simulink model "Controller_CalDistance0"  (R2020b)
settings: Solver=FixedStepDiscrete  StartTime=0.0  StopTime=inf  FixedStep=1e-06  RelTol=1e-3  EnableMultiTasking=on
settings Model: SILPILModeSetting=veronly  ExtModeTrigDuration=2  Creator=99714  LastModifiedBy=99714
settings DataIOCC: SaveOutput=off  SaveTime=off
settings OptimizationCC: EnhancedBackFolding=on  PassReuseOutputArgsAs=Individual arguments  MaxStackSize=64  OptimizeBlockOrder=speed  DifferentSizesBufferReuse=on  OptimizationCustomize=off  EfficientTunableParamExpr=on
settings DebuggingCC: ParameterTunabilityLossMsg=error
settings HardwareCC: ProdBitPerInt=16  ProdBitPerPointer=16  ProdBitPerSizeT=16  ProdBitPerPtrDiffT=16  ProdLargestAtomicFloat=None  ProdWordSize=8  ProdHWDeviceType=Atmel->AVR
settings SFSimCC: MATLABDynamicMemAlloc=off
settings RTWCC: Description=Embedded Coder  SystemTargetFile=ert.tlc  HardwareBoard=Arduino Uno  GenCodeOnly=on  TemplateMakefile=ert_default_tmf  GenerateReport=on  Toolchain=Arduino AVR  BuildConfiguration=Faster Runs  IncludeHyperlinkInReport=on  LaunchReport=on  GenerateWebview=on  GenerateCodeMetricsReport=on
settings CodeAppCC: ForceParamTrailComments=on  IgnoreCustomStorageClasses=off  OperatorAnnotations=on  SimulinkDataObjDesc=on  SFDataObjDesc=on  InsertBlockDesc=on
settings ERTTargetCC: CodeInterfacePackaging=Reusable function  SupportContinuousTime=on  SupportVariableSizeSignals=on  ExtModeStaticAllocSize=250
settings ConfigComp: CovEnable=on  CovScope=Subsystem  RecordCoverage=on  CovEnableCumulative=off  CovSaveSingleToWorkspaceVar=on  CovExternalEMLEnable=off  CovSFcnEnable=off

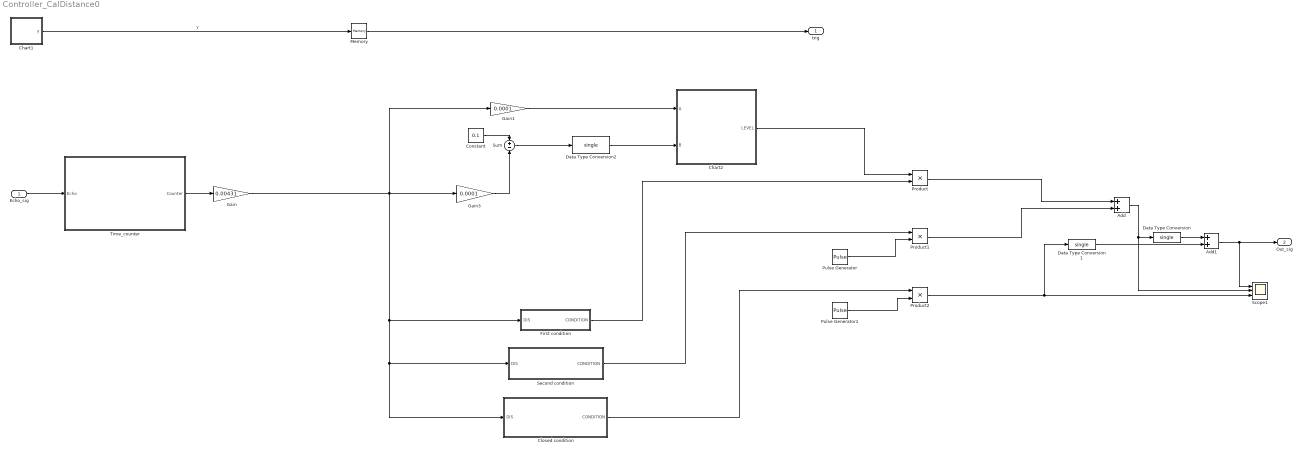
== system Controller_CalDistance0 ==
  Echo_sig : Inport  OutDataTypeStr=single  PortDimensions=1
  Add : Sum
  Add1 : Sum
  Chart1 : Stateflow chart  TreatAsAtomicUnit=on
  Chart2 : Stateflow chart  TreatAsAtomicUnit=on
  Closed condition : Stateflow chart  TreatAsAtomicUnit=on
  Constant : Constant  Value=0.1
  Data Type Conversion : DataTypeConversion  OutDataTypeStr=single
  Data Type Conversion1 : DataTypeConversion  OutDataTypeStr=single
  Data Type Conversion2 : DataTypeConversion  OutDataTypeStr=single
  First condition : Stateflow chart  TreatAsAtomicUnit=on
  Gain : Gain  Gain=0.00431
  Gain1 : Gain  Gain=0.0001
  Gain3 : Gain  Gain=0.0001
  Memory : Memory  InitialCondition=1  InheritSampleTime=on  LinearizeMemory=on
  Product : Product
  Product1 : Product
  Product2 : Product
  Pulse Generator : DiscretePulseGenerator  PulseType=Time based  Period=0.5  PulseWidth=50
  Pulse Generator1 : DiscretePulseGenerator  PulseType=Time based  Period=1  PulseWidth=50
  Scope1 : Scope  NumInputPorts=3
  Second condition : Stateflow chart  TreatAsAtomicUnit=on
  Sum : Sum  Inputs=+-
  Time_counter : Stateflow chart  TreatAsAtomicUnit=on
  trig : Outport  OutDataTypeStr=single  PortDimensions=1  SampleTime=[9.9999999999999995e-07,0]
  Out_sig : Outport  Port=2  OutDataTypeStr=single  PortDimensions=1  SampleTime=[9.9999999999999995e-07,0]
  wires:
  Chart1/1(y) -> Memory/1  "y"
  Echo_sig/1 -> Time_counter/1(Echo)
  Time_counter/1(Counter) -> Gain/1
  Product/1 -> Add/1
  Pulse Generator/1 -> Product1/2
  Pulse Generator1/1 -> Product2/2
  Add/1 -> Scope1/2, Data Type Conversion/1
  Memory/1 -> trig/1
  Data Type Conversion2/1 -> Chart2/2(B)
  Sum/1 -> Data Type Conversion2/1
  Gain1/1 -> Chart2/1(A)
  Gain3/1 -> Sum/2
  Constant/1 -> Sum/1
  First condition/1(CONDITION) -> Product/2
  Second condition/1(CONDITION) -> Product1/1
  Closed condition/1(CONDITION) -> Product2/1
  Chart2/1(LEVEL) -> Product/1
  Product1/1 -> Add/2
  Product2/1 -> Scope1/3, Data Type Conversion1/1
  Add1/1 -> Scope1/1, Out_sig/1
  Data Type Conversion/1 -> Add1/1
  Data Type Conversion1/1 -> Add1/2
  Gain/1 -> Closed condition/1(DIS), Second condition/1(DIS), First condition/1(DIS), Gain3/1, Gain1/1

== stateflow chart Controller_CalDistance0/First condition ==
  state WAIT
  state STANE_BY
    en:CONDITION=0;
  state CONFIRM
    en:CONDITION=1;
  (default) -> WAIT
  WAIT -> STANE_BY : after(0.1,sec)
  STANE_BY -> CONFIRM : [DIS>=10&&DIS<100]
  data: CONDITION output single; DIS input single

== stateflow chart Controller_CalDistance0/Chart2 ==
  state LEVEL_1_ON
    state START
      en:LEVEL=1
    state OFF
      en:LEVEL=0
    (default) -> START
    START -> OFF : [after(A,sec)]
    OFF -> START : [after(B,sec)]
  (default) -> LEVEL_1_ON
  data: A input single; LEVEL output single; B input single

== stateflow chart Controller_CalDistance0/Second condition ==
  state WAIT
  state STAND_BY
    en:CONDITION=0;
  state CINFIRM
    en:CONDITION=1;
  (default) -> WAIT
  WAIT -> STAND_BY : after(0.2,sec)
  STAND_BY -> CINFIRM : [DIS>0&&DIS<10||DIS>100]
  data: DIS input single; CONDITION output single

== stateflow chart Controller_CalDistance0/Chart1 ==
  state Trig_On
    en:y=1
  state Trig_Off
    en:y=0
  (default) -> Trig_On
  Trig_Off -> Trig_On : after(60,msec)
  Trig_On -> Trig_Off : after(10,usec)
  data: y output single

== stateflow chart Controller_CalDistance0/Closed condition ==
  state SATND_BY
  state CHECK
  state CONFIRM
    en:CONDITION=1;
  (default) -> SATND_BY
  SATND_BY -> CHECK : [after(0.07,sec)]
  CHECK -> CONFIRM : [DIS==0]
  data: CONDITION output single; DIS input single

== stateflow chart Controller_CalDistance0/Time_counter ==
  state Initiation
    en:Timer=0;
    Counter=0;
  state Stand_by
    en:Timer=Timer+1;
  state ON
    du:Counter=Counter+1;
  state OFF
  (default) -> Initiation
  Initiation -> Stand_by
  OFF -> Stand_by : [Timer<4]
  Stand_by -> ON : [Echo==1]
  ON -> OFF : [Echo==0]
  data: Echo input single; Timer local single; Counter output single
